simulink model "bicyclemodel_step_disturbance_force"  (R2020b)
settings: Solver=ode5  StartTime=0.0  StopTime=tf  FixedStep=dt  RelTol=1e-3
values from neighbouring files (symbols this model uses):
  I = 2500    [bicyclemodle_setp_disturbance_force_Param.m]    (also in bicyclemodle_stepParam.m; twoDOFmodel_side_wind_gust_Param.m)
  Kf = 55000    [bicyclemodle_setp_disturbance_force_Param.m]    (also in bicyclemodle_stepParam.m; twoDOFmodel_side_wind_gust_Param.m)
  lf = 1.1    [bicyclemodle_setp_disturbance_force_Param.m]    (also in bicyclemodle_stepParam.m; twoDOFmodel_side_wind_gust_Param.m)
  m = 1500    [bicyclemodle_setp_disturbance_force_Param.m]    (also in bicyclemodle_stepParam.m; twoDOFmodel_side_wind_gust_Param.m)
  Sf = 0.0    (= 0)    [bicyclemodle_setp_disturbance_force_Param.m]    (also in bicyclemodle_stepParam.m = 0.04; twoDOFmodel_side_wind_gust_Param.m)
  V = 80/3.6    (= 22.2222222222)    [bicyclemodle_setp_disturbance_force_Param.m]    (also in bicyclemodle_stepParam.m = 38.8888888889; twoDOFmodel_side_wind_gust_Param.m = 40)
  Y0 = 4000    [bicyclemodle_setp_disturbance_force_Param.m]
libraries: simulink x1
settings Model: Creator=Anson  LastModifiedBy=Anson

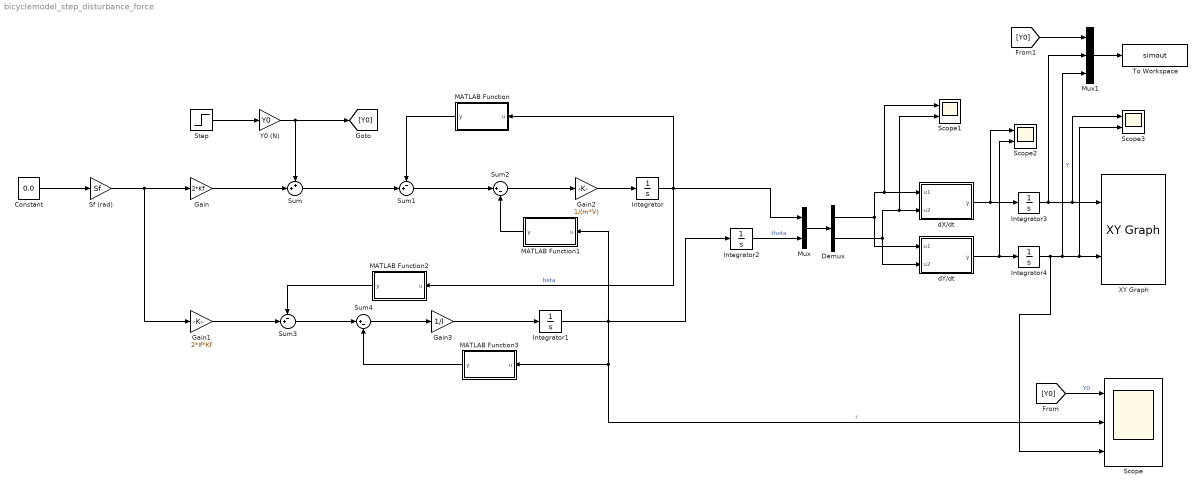
== system bicyclemodel_step_disturbance_force ==
  Constant : Constant  Value=0.0
  Demux : Demux  Outputs=2
  Gain : Gain  Gain=2*Kf
  Gain1 : Gain  Gain=2*lf*Kf
  Gain2 : Gain  Gain=1/(m*V)
  Gain3 : Gain  Gain=1/I
  Integrator{,1..4} (5 alike) : Integrator
  MATLAB Function : MATLAB Function  TreatAsAtomicUnit=on
  MATLAB Function1 : MATLAB Function  TreatAsAtomicUnit=on
  MATLAB Function2 : MATLAB Function  TreatAsAtomicUnit=on
  MATLAB Function3 : MATLAB Function  TreatAsAtomicUnit=on
  Mux : Mux  Inputs=2
  Mux1 : Mux  Inputs=3
  Scope : Scope  NumInputPorts=3
  Scope1 : Scope  NumInputPorts=2
  Scope2 : Scope  NumInputPorts=2
  Scope3 : Scope  NumInputPorts=2
  Sf (rad) : Gain  Gain=Sf
  Step : Step  Time=0.5  SampleTime=0
  Sum : Sum  Inputs=++|
  Sum1 : Sum  Inputs=-+|
  Sum2 : Sum  Inputs=|+-
  Sum3 : Sum  Inputs=-+|
  Sum4 : Sum  Inputs=|+-
  To Workspace : ToWorkspace  VariableName=simout  SaveFormat=Timeseries  SampleTime=-1
  XY Graph : simulink/Sinks/XY Graph  xmin=-1  xmax=90  ymin=-1  ymax=10  st=-1
  Y0 (N) : Gain  Gain=Y0
  dX/dt : MATLAB Function  TreatAsAtomicUnit=on
  dY/dt : MATLAB Function  TreatAsAtomicUnit=on
  wires:
  Constant/1 -> Sf (rad)/1
  Sf (rad)/1 -> Gain1/1, Gain/1
  Gain/1 -> Sum/2
  Step/1 -> Y0 (N)/1
  Y0 (N)/1 -> [Y0], Sum/1
  Sum/1 -> Sum1/2
  MATLAB Function/1(y) -> Sum1/1
  Sum1/1 -> Sum2/1
  Sum2/1 -> Gain2/1
  MATLAB Function1/1(y) -> Sum2/2
  Gain2/1 -> Integrator/1
  Integrator/1 -> MATLAB Function2/1(u), Mux/1, MATLAB Function/1(u)  "beta"
  Gain1/1 -> Sum3/2
  Sum3/1 -> Sum4/1
  MATLAB Function2/1(y) -> Sum3/1
  MATLAB Function3/1(y) -> Sum4/2
  Sum4/1 -> Gain3/1
  Gain3/1 -> Integrator1/1
  Integrator1/1 -> Scope/2, MATLAB Function3/1(u), MATLAB Function1/1(u), Integrator2/1  "r"
  Integrator2/1 -> Mux/2  "theta"
  Mux/1 -> Demux/1
  Demux/1 -> dY/dt/1(u1), Scope1/1, dX/dt/1(u1)
  Demux/2 -> dY/dt/2(u2), Scope1/2, dX/dt/2(u2)
  dX/dt/1(y) -> Scope2/1, Integrator3/1
  dY/dt/1(y) -> Scope2/2, Integrator4/1
  Integrator3/1 -> Mux1/2, Scope3/1, XY Graph/1
  Integrator4/1 -> Mux1/3, Scope3/2, XY Graph/2, Scope/3  "Y"
  Mux1/1 -> To Workspace/1
  [Y0] -> Mux1/1
  [Y0] -> Scope/1  "Y0"

== matlab function bicyclemodel_step_disturbance_force/MATLAB Function ==
  data: u input; y output
function y = fcn(u)
Kf = 55000;% front cornering stiffness (N/rad)
Kr = 60000;% rear cornering stiffness (N/rad)
y = 2*(Kf+Kr)*u;

== matlab function bicyclemodel_step_disturbance_force/MATLAB Function2 ==
  data: u input; y output
function y = fcn(u)
lf = 1.1;       % distance from C.O.C to front axle (m)
lr = 1.6;       % distance from C.O.C to rear axle (m)
Kf = 55000;% front cornering stiffness (N/rad)
Kr = 60000;% rear cornering stiffness (N/rad)
y = (2*(lf*Kf-lr*Kr))*u;

== matlab function bicyclemodel_step_disturbance_force/MATLAB Function3 ==
  data: u input; y output
function y = fcn(u)
lf = 1.1;       % distance from C.O.C to front axle (m)
lr = 1.6;       % distance from C.O.C to rear axle (m)
V = 80/3.6; % velocity (m/s)
Kf = 55000;% front cornering stiffness (N/rad)
Kr = 60000;% rear cornering stiffness (N/rad)
y = (2*(lf*lf*Kf+lr*lr*Kr)/V)*u;

== matlab function bicyclemodel_step_disturbance_force/dX//dt ==
  data: u1 input; y output; u2 input
function y = fcn(u1, u2)
V = 80/3.6; % velocity (m/s)
y = V*cos(u1+u2);

== matlab function bicyclemodel_step_disturbance_force/dY//dt ==
  data: u1 input; y output; u2 input
function y = fcn(u1, u2)
V = 80/3.6; % velocity (m/s)
y = V*sin(u1+u2);

== matlab function bicyclemodel_step_disturbance_force/MATLAB Function1 ==
  data: u input; y output
function y = fcn(u)
m = 1500;   % mass (kg)
V = 80/3.6; % velocity (m/s)
lf = 1.1;       % distance from C.O.C to front axle (m)
lr = 1.6;       % distance from C.O.C to rear axle (m)
Kf = 55000;% front cornering stiffness (N/rad)
Kr = 60000;% rear cornering stiffness (N/rad)
y = ((m*V)+2*(lf*Kf-lr*Kr)/V)*u;
